simulink model "untitled"  (R2017a)
settings: Solver=FixedStepAuto  StartTime=0.0  StopTime=inf  FixedStep=0.1  RelTol=1e-3
settings Model: Creator=guo  LastModifiedBy=guo

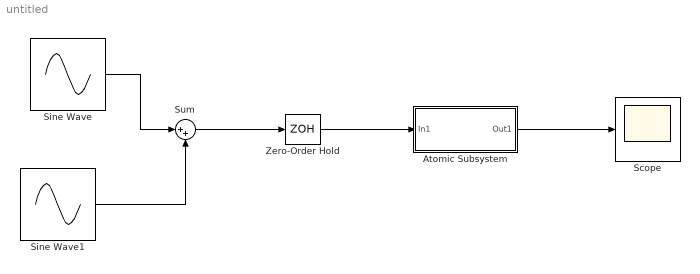
== system untitled ==
  Atomic Subsystem : Subsystem  TreatAsAtomicUnit=on
  Scope : Scope
  Sine Wave : Sin  Frequency=500  SampleTime=0
  Sine Wave1 : Sin  Frequency=3000  SampleTime=0
  Sum : Sum  Inputs=|++
  Zero-Order Hold : ZeroOrderHold  SampleTime=-1
  wires:
  Sine Wave/1 -> Sum/1
  Sine Wave1/1 -> Sum/2
  Sum/1 -> Zero-Order Hold/1
  Zero-Order Hold/1 -> Atomic Subsystem/1(In1)
  Atomic Subsystem/1(Out1) -> Scope/1

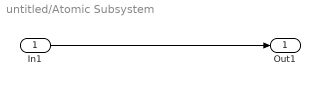
== system untitled/Atomic Subsystem ==
  In1 : Inport
  Out1 : Outport
  wires:
  In1/1 -> Out1/1
